simulink model "armModelLQG"  (R2018b)
settings: Solver=ode15s  StartTime=0.0  StopTime=10  MaxStep=1e-4  RelTol=1e-6  AbsTol=1e-7
values from neighbouring files (symbols this model uses):
  Cv1 = 1.3*10^(-6)*60/(2*pi)    (= 1.24140855612e-05)    [setup.m]
  Cv2 = 1.3*10^(-6)*60/(2*pi)    (= 1.24140855612e-05)    [setup.m]
  Cv3 = 1.3*10^(-6)*60/(2*pi)    (= 1.24140855612e-05)    [setup.m]
  effWorm = 0.8    [setup.m]
  J1 = 1.3*10^(-4)    (= 0.00013)    [setup.m]
  J2 = 0.79*10^(-4)    (= 7.9e-05)    [setup.m]
  J3 = 0.98*10^(-4)    (= 9.8e-05)    [setup.m]
  Ke1 = 0.15    [setup.m]
  Ke2 = 0.12    [setup.m]
  Ke3 = 0.12    [setup.m]
  Km1 = 0.15    [setup.m]
  Km2 = 0.12    [setup.m]
  Km3 = 0.12    [setup.m]
  N1 = 36    [setup.m]
  N2 = 36    [setup.m]
  N3 = 36    [setup.m]
  R1 = 1.9    [setup.m]
  R2 = 2.45    [setup.m]
  R3 = 1.9    [setup.m]
undefined symbols (not defined in the file or in its folder): A, B, C, Continuous, D, Time, X, Y, Z
libraries: sm_lib x92, nesl_utility x26, simulink x5, Parts_Lib x2, Contact_Forces_Lib x2, ctrlSharedLib x1
(part 4 of 4)

== system armModelLQG/ARM plant /Pop Transform4 1 ==
  Rotational fix1 : sm_lib/Frames and Transforms/Rigid Transform  TranslationMethod=None  TranslationStandardOffset=0  TranslationLengthUnit=m  TranslationStandardAxis=+Z  TranslationCartesianOffset=[0 0 0]  TranslationROffset=0  TranslationROffsetUnits=m  TranslationZOffset=0  TranslationZOffsetUnits=m  TranslationThetaOffset=0  TranslationThetaOffsetUnits=deg  RotationMethod=StandardAxis  RotationAngleUnits=deg  RotationStandardAxis=-Y  RotationAngle=90  RotationArbitraryAxis=[0 0 1]  FollAlignAxisA=+X  BaseAlignAxisA=+Y  FollAlignAxisB=+Y  BaseAlignAxisB=+Z  RotationSequenceAxes=FollowerAxes  RotationSequence=XYX  RotationSequenceAngles=[0 0 0]  RotationSequenceAnglesUnits=deg  RotationMatrix=[1 0 0; 0 1 0; 0 0 1]
  Rotational fix2 : sm_lib/Frames and Transforms/Rigid Transform  TranslationMethod=None  TranslationStandardOffset=0  TranslationLengthUnit=m  TranslationStandardAxis=+Z  TranslationCartesianOffset=[0 0 0]  TranslationROffset=0  TranslationROffsetUnits=m  TranslationZOffset=0  TranslationZOffsetUnits=m  TranslationThetaOffset=0  TranslationThetaOffsetUnits=deg  RotationMethod=StandardAxis  RotationAngleUnits=deg  RotationStandardAxis=-X  RotationAngle=90  RotationArbitraryAxis=[0 0 1]  FollAlignAxisA=+X  BaseAlignAxisA=+Y  FollAlignAxisB=+Y  BaseAlignAxisB=+Z  RotationSequenceAxes=FollowerAxes  RotationSequence=XYX  RotationSequenceAngles=[0 0 0]  RotationSequenceAnglesUnits=deg  RotationMatrix=[1 0 0; 0 1 0; 0 0 1]
  "Transform X " : sm_lib/Frames and Transforms/Rigid Transform  TranslationMethod=StandardAxis  TranslationStandardOffset=67.6  TranslationLengthUnit=mm  TranslationStandardAxis=-X  TranslationCartesianOffset=[0 0 -188]  TranslationROffset=0  TranslationROffsetUnits=m  TranslationZOffset=0  TranslationZOffsetUnits=m  TranslationThetaOffset=0  TranslationThetaOffsetUnits=deg  RotationMethod=None  RotationAngleUnits=deg  RotationStandardAxis=+Y  RotationAngle=90  RotationArbitraryAxis=[0 0 1]  FollAlignAxisA=+X  BaseAlignAxisA=+Y  FollAlignAxisB=+Y  BaseAlignAxisB=+Z  RotationSequenceAxes=FollowerAxes  RotationSequence=XYX  RotationSequenceAngles=[0 0 0]  RotationSequenceAnglesUnits=deg  RotationMatrix=[1 0 0; 0 1 0; 0 0 1]
  Transform y : sm_lib/Frames and Transforms/Rigid Transform  TranslationMethod=StandardAxis  TranslationStandardOffset=-447.93  TranslationLengthUnit=mm  TranslationStandardAxis=-Y  TranslationCartesianOffset=[0 0 -188]  TranslationROffset=0  TranslationROffsetUnits=m  TranslationZOffset=0  TranslationZOffsetUnits=m  TranslationThetaOffset=0  TranslationThetaOffsetUnits=deg  RotationMethod=None  RotationAngleUnits=deg  RotationStandardAxis=+Y  RotationAngle=90  RotationArbitraryAxis=[0 0 1]  FollAlignAxisA=+X  BaseAlignAxisA=+Y  FollAlignAxisB=+Y  BaseAlignAxisB=+Z  RotationSequenceAxes=FollowerAxes  RotationSequence=XYX  RotationSequenceAngles=[0 0 0]  RotationSequenceAnglesUnits=deg  RotationMatrix=[1 0 0; 0 1 0; 0 0 1]
  Transform z : sm_lib/Frames and Transforms/Rigid Transform  TranslationMethod=StandardAxis  TranslationStandardOffset=0.59  TranslationLengthUnit=mm  TranslationStandardAxis=-Z  TranslationCartesianOffset=[0 0 -188]  TranslationROffset=0  TranslationROffsetUnits=m  TranslationZOffset=0  TranslationZOffsetUnits=m  TranslationThetaOffset=0  TranslationThetaOffsetUnits=deg  RotationMethod=None  RotationAngleUnits=deg  RotationStandardAxis=+Y  RotationAngle=90  RotationArbitraryAxis=[0 0 1]  FollAlignAxisA=+X  BaseAlignAxisA=+Y  FollAlignAxisB=+Y  BaseAlignAxisB=+Z  RotationSequenceAxes=FollowerAxes  RotationSequence=XYX  RotationSequenceAngles=[0 0 0]  RotationSequenceAnglesUnits=deg  RotationMatrix=[1 0 0; 0 1 0; 0 0 1]
  Conn1 : PMIOPort  Side=Left
  Conn2 : PMIOPort  Port=2  Side=Right
  connections:
  Rotational fix1/RConn1 -- Conn2/RConn1
  Transform z/RConn1 -- Rotational fix1/LConn1
  Rotational fix2/RConn1 -- "Transform X "/LConn1
  Transform y/LConn1 -- "Transform X "/RConn1
  Transform z/LConn1 -- Transform y/RConn1
  Conn1/RConn1 -- Rotational fix2/LConn1

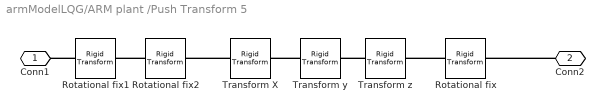
== system armModelLQG/ARM plant /Push Transform 5 ==
  Rotational fix : sm_lib/Frames and Transforms/Rigid Transform  TranslationMethod=None  TranslationStandardOffset=0  TranslationLengthUnit=m  TranslationStandardAxis=+Z  TranslationCartesianOffset=[0 0 0]  TranslationROffset=0  TranslationROffsetUnits=m  TranslationZOffset=0  TranslationZOffsetUnits=m  TranslationThetaOffset=0  TranslationThetaOffsetUnits=deg  RotationMethod=StandardAxis  RotationAngleUnits=deg  RotationStandardAxis=+X  RotationAngle=90  RotationArbitraryAxis=[0 0 1]  FollAlignAxisA=+X  BaseAlignAxisA=+Y  FollAlignAxisB=+Y  BaseAlignAxisB=+Z  RotationSequenceAxes=FollowerAxes  RotationSequence=XYX  RotationSequenceAngles=[0 0 0]  RotationSequenceAnglesUnits=deg  RotationMatrix=[1 0 0; 0 1 0; 0 0 1]
  Rotational fix1 : sm_lib/Frames and Transforms/Rigid Transform  TranslationMethod=None  TranslationStandardOffset=0  TranslationLengthUnit=m  TranslationStandardAxis=+Z  TranslationCartesianOffset=[0 0 0]  TranslationROffset=0  TranslationROffsetUnits=m  TranslationZOffset=0  TranslationZOffsetUnits=m  TranslationThetaOffset=0  TranslationThetaOffsetUnits=deg  RotationMethod=StandardAxis  RotationAngleUnits=deg  RotationStandardAxis=+Y  RotationAngle=-90  RotationArbitraryAxis=[0 0 1]  FollAlignAxisA=+X  BaseAlignAxisA=+Y  FollAlignAxisB=+Y  BaseAlignAxisB=+Z  RotationSequenceAxes=FollowerAxes  RotationSequence=XYX  RotationSequenceAngles=[0 0 0]  RotationSequenceAnglesUnits=deg  RotationMatrix=[1 0 0; 0 1 0; 0 0 1]
  Rotational fix2 : sm_lib/Frames and Transforms/Rigid Transform  TranslationMethod=None  TranslationStandardOffset=0  TranslationLengthUnit=m  TranslationStandardAxis=+Z  TranslationCartesianOffset=[0 0 0]  TranslationROffset=0  TranslationROffsetUnits=m  TranslationZOffset=0  TranslationZOffsetUnits=m  TranslationThetaOffset=0  TranslationThetaOffsetUnits=deg  RotationMethod=StandardAxis  RotationAngleUnits=deg  RotationStandardAxis=+X  RotationAngle=0  RotationArbitraryAxis=[0 0 1]  FollAlignAxisA=+X  BaseAlignAxisA=+Y  FollAlignAxisB=+Y  BaseAlignAxisB=+Z  RotationSequenceAxes=FollowerAxes  RotationSequence=XYX  RotationSequenceAngles=[0 0 0]  RotationSequenceAnglesUnits=deg  RotationMatrix=[1 0 0; 0 1 0; 0 0 1]
  "Transform X " : sm_lib/Frames and Transforms/Rigid Transform  TranslationMethod=StandardAxis  TranslationStandardOffset=18.98  TranslationLengthUnit=mm  TranslationStandardAxis=+X  TranslationCartesianOffset=[0 0 -188]  TranslationROffset=0  TranslationROffsetUnits=m  TranslationZOffset=0  TranslationZOffsetUnits=m  TranslationThetaOffset=0  TranslationThetaOffsetUnits=deg  RotationMethod=None  RotationAngleUnits=deg  RotationStandardAxis=+Y  RotationAngle=90  RotationArbitraryAxis=[0 0 1]  FollAlignAxisA=+X  BaseAlignAxisA=+Y  FollAlignAxisB=+Y  BaseAlignAxisB=+Z  RotationSequenceAxes=FollowerAxes  RotationSequence=XYX  RotationSequenceAngles=[0 0 0]  RotationSequenceAnglesUnits=deg  RotationMatrix=[1 0 0; 0 1 0; 0 0 1]
  Transform y : sm_lib/Frames and Transforms/Rigid Transform  TranslationMethod=StandardAxis  TranslationStandardOffset=-11.18  TranslationLengthUnit=mm  TranslationStandardAxis=+Y  TranslationCartesianOffset=[0 0 -188]  TranslationROffset=0  TranslationROffsetUnits=m  TranslationZOffset=0  TranslationZOffsetUnits=m  TranslationThetaOffset=0  TranslationThetaOffsetUnits=deg  RotationMethod=None  RotationAngleUnits=deg  RotationStandardAxis=+Y  RotationAngle=90  RotationArbitraryAxis=[0 0 1]  FollAlignAxisA=+X  BaseAlignAxisA=+Y  FollAlignAxisB=+Y  BaseAlignAxisB=+Z  RotationSequenceAxes=FollowerAxes  RotationSequence=XYX  RotationSequenceAngles=[0 0 0]  RotationSequenceAnglesUnits=deg  RotationMatrix=[1 0 0; 0 1 0; 0 0 1]
  Transform z : sm_lib/Frames and Transforms/Rigid Transform  TranslationMethod=StandardAxis  TranslationStandardOffset=-10  TranslationLengthUnit=mm  TranslationStandardAxis=+Z  TranslationCartesianOffset=[0 0 -188]  TranslationROffset=0  TranslationROffsetUnits=m  TranslationZOffset=0  TranslationZOffsetUnits=m  TranslationThetaOffset=0  TranslationThetaOffsetUnits=deg  RotationMethod=None  RotationAngleUnits=deg  RotationStandardAxis=+Y  RotationAngle=90  RotationArbitraryAxis=[0 0 1]  FollAlignAxisA=+X  BaseAlignAxisA=+Y  FollAlignAxisB=+Y  BaseAlignAxisB=+Z  RotationSequenceAxes=FollowerAxes  RotationSequence=XYX  RotationSequenceAngles=[0 0 0]  RotationSequenceAnglesUnits=deg  RotationMatrix=[1 0 0; 0 1 0; 0 0 1]
  Conn1 : PMIOPort  Side=Left
  Conn2 : PMIOPort  Port=2  Side=Right
  connections:
  Conn2/RConn1 -- Rotational fix/RConn1
  Rotational fix/LConn1 -- Transform z/RConn1
  "Transform X "/LConn1 -- Rotational fix2/RConn1
  Transform y/LConn1 -- "Transform X "/RConn1
  Transform z/LConn1 -- Transform y/RConn1
  Rotational fix1/LConn1 -- Conn1/RConn1
  Rotational fix2/LConn1 -- Rotational fix1/RConn1

== system armModelLQG/ARM plant /Push Transform1  ==
  Rotational fix : sm_lib/Frames and Transforms/Rigid Transform  TranslationMethod=None  TranslationStandardOffset=0  TranslationLengthUnit=m  TranslationStandardAxis=+Z  TranslationCartesianOffset=[0 0 0]  TranslationROffset=0  TranslationROffsetUnits=m  TranslationZOffset=0  TranslationZOffsetUnits=m  TranslationThetaOffset=0  TranslationThetaOffsetUnits=deg  RotationMethod=StandardAxis  RotationAngleUnits=deg  RotationStandardAxis=+Y  RotationAngle=-90  RotationArbitraryAxis=[0 0 1]  FollAlignAxisA=+X  BaseAlignAxisA=+Y  FollAlignAxisB=+Y  BaseAlignAxisB=+Z  RotationSequenceAxes=FollowerAxes  RotationSequence=XYX  RotationSequenceAngles=[0 0 0]  RotationSequenceAnglesUnits=deg  RotationMatrix=[1 0 0; 0 1 0; 0 0 1]
  "Transform Y 1 " : sm_lib/Frames and Transforms/Rigid Transform  TranslationMethod=StandardAxis  TranslationStandardOffset=-29  TranslationLengthUnit=mm  TranslationStandardAxis=+Y  TranslationCartesianOffset=[0 0 0]  TranslationROffset=0  TranslationROffsetUnits=m  TranslationZOffset=0  TranslationZOffsetUnits=m  TranslationThetaOffset=0  TranslationThetaOffsetUnits=deg  RotationMethod=None  RotationAngleUnits=deg  RotationStandardAxis=+Y  RotationAngle=90  RotationArbitraryAxis=[0 0 1]  FollAlignAxisA=+X  BaseAlignAxisA=+Y  FollAlignAxisB=+Y  BaseAlignAxisB=+Z  RotationSequenceAxes=FollowerAxes  RotationSequence=XYX  RotationSequenceAngles=[0 0 0]  RotationSequenceAnglesUnits=deg  RotationMatrix=[1 0 0; 0 1 0; 0 0 1]
  "Transform Z 1 " : sm_lib/Frames and Transforms/Rigid Transform  TranslationMethod=StandardAxis  TranslationStandardOffset=-32  TranslationLengthUnit=mm  TranslationStandardAxis=+Z  TranslationCartesianOffset=[0 0 0]  TranslationROffset=0  TranslationROffsetUnits=m  TranslationZOffset=0  TranslationZOffsetUnits=m  TranslationThetaOffset=0  TranslationThetaOffsetUnits=deg  RotationMethod=None  RotationAngleUnits=deg  RotationStandardAxis=+Y  RotationAngle=90  RotationArbitraryAxis=[0 0 1]  FollAlignAxisA=+X  BaseAlignAxisA=+Y  FollAlignAxisB=+Y  BaseAlignAxisB=+Z  RotationSequenceAxes=FollowerAxes  RotationSequence=XYX  RotationSequenceAngles=[0 0 0]  RotationSequenceAnglesUnits=deg  RotationMatrix=[1 0 0; 0 1 0; 0 0 1]
  Conn1 : PMIOPort  Side=Left
  Conn2 : PMIOPort  Port=2  Side=Right
  connections:
  "Transform Z 1 "/LConn1 -- "Transform Y 1 "/RConn1
  Conn2/RConn1 -- Rotational fix/RConn1
  Rotational fix/LConn1 -- "Transform Z 1 "/RConn1
  Conn1/RConn1 -- "Transform Y 1 "/LConn1

== system armModelLQG/ARM plant /Push Transform2  ==
  Rotational fix : sm_lib/Frames and Transforms/Rigid Transform  TranslationMethod=None  TranslationStandardOffset=0  TranslationLengthUnit=m  TranslationStandardAxis=+Z  TranslationCartesianOffset=[0 0 0]  TranslationROffset=0  TranslationROffsetUnits=m  TranslationZOffset=0  TranslationZOffsetUnits=m  TranslationThetaOffset=0  TranslationThetaOffsetUnits=deg  RotationMethod=StandardAxis  RotationAngleUnits=deg  RotationStandardAxis=+Y  RotationAngle=90  RotationArbitraryAxis=[0 0 1]  FollAlignAxisA=+X  BaseAlignAxisA=+Y  FollAlignAxisB=+Y  BaseAlignAxisB=+Z  RotationSequenceAxes=FollowerAxes  RotationSequence=XYX  RotationSequenceAngles=[0 0 0]  RotationSequenceAnglesUnits=deg  RotationMatrix=[1 0 0; 0 1 0; 0 0 1]
  "Transform X " : sm_lib/Frames and Transforms/Rigid Transform  TranslationMethod=StandardAxis  TranslationStandardOffset=-188  TranslationLengthUnit=mm  TranslationStandardAxis=+X  TranslationCartesianOffset=[0 0 -188]  TranslationROffset=0  TranslationROffsetUnits=m  TranslationZOffset=0  TranslationZOffsetUnits=m  TranslationThetaOffset=0  TranslationThetaOffsetUnits=deg  RotationMethod=None  RotationAngleUnits=deg  RotationStandardAxis=+Y  RotationAngle=90  RotationArbitraryAxis=[0 0 1]  FollAlignAxisA=+X  BaseAlignAxisA=+Y  FollAlignAxisB=+Y  BaseAlignAxisB=+Z  RotationSequenceAxes=FollowerAxes  RotationSequence=XYX  RotationSequenceAngles=[0 0 0]  RotationSequenceAnglesUnits=deg  RotationMatrix=[1 0 0; 0 1 0; 0 0 1]
  Conn1 : PMIOPort  Side=Left
  Conn2 : PMIOPort  Port=2  Side=Right
  connections:
  Conn2/RConn1 -- Rotational fix/RConn1
  Rotational fix/LConn1 -- "Transform X "/RConn1
  "Transform X "/LConn1 -- Conn1/RConn1

== system armModelLQG/ARM plant /Push Transform3  ==
  Rotational fix : sm_lib/Frames and Transforms/Rigid Transform  TranslationMethod=None  TranslationStandardOffset=0  TranslationLengthUnit=m  TranslationStandardAxis=+Z  TranslationCartesianOffset=[0 0 0]  TranslationROffset=0  TranslationROffsetUnits=m  TranslationZOffset=0  TranslationZOffsetUnits=m  TranslationThetaOffset=0  TranslationThetaOffsetUnits=deg  RotationMethod=StandardAxis  RotationAngleUnits=deg  RotationStandardAxis=+Y  RotationAngle=-90  RotationArbitraryAxis=[0 0 1]  FollAlignAxisA=+X  BaseAlignAxisA=+Y  FollAlignAxisB=+Y  BaseAlignAxisB=+Z  RotationSequenceAxes=FollowerAxes  RotationSequence=XYX  RotationSequenceAngles=[0 0 0]  RotationSequenceAnglesUnits=deg  RotationMatrix=[1 0 0; 0 1 0; 0 0 1]
  "Transform X " : sm_lib/Frames and Transforms/Rigid Transform  TranslationMethod=StandardAxis  TranslationStandardOffset=20  TranslationLengthUnit=mm  TranslationStandardAxis=+X  TranslationCartesianOffset=[0 0 -188]  TranslationROffset=0  TranslationROffsetUnits=m  TranslationZOffset=0  TranslationZOffsetUnits=m  TranslationThetaOffset=0  TranslationThetaOffsetUnits=deg  RotationMethod=None  RotationAngleUnits=deg  RotationStandardAxis=+Y  RotationAngle=90  RotationArbitraryAxis=[0 0 1]  FollAlignAxisA=+X  BaseAlignAxisA=+Y  FollAlignAxisB=+Y  BaseAlignAxisB=+Z  RotationSequenceAxes=FollowerAxes  RotationSequence=XYX  RotationSequenceAngles=[0 0 0]  RotationSequenceAnglesUnits=deg  RotationMatrix=[1 0 0; 0 1 0; 0 0 1]
  Transform y : sm_lib/Frames and Transforms/Rigid Transform  TranslationMethod=StandardAxis  TranslationStandardOffset=-0.22  TranslationLengthUnit=mm  TranslationStandardAxis=+Y  TranslationCartesianOffset=[0 0 -188]  TranslationROffset=0  TranslationROffsetUnits=m  TranslationZOffset=0  TranslationZOffsetUnits=m  TranslationThetaOffset=0  TranslationThetaOffsetUnits=deg  RotationMethod=None  RotationAngleUnits=deg  RotationStandardAxis=+Y  RotationAngle=90  RotationArbitraryAxis=[0 0 1]  FollAlignAxisA=+X  BaseAlignAxisA=+Y  FollAlignAxisB=+Y  BaseAlignAxisB=+Z  RotationSequenceAxes=FollowerAxes  RotationSequence=XYX  RotationSequenceAngles=[0 0 0]  RotationSequenceAnglesUnits=deg  RotationMatrix=[1 0 0; 0 1 0; 0 0 1]
  Transform z : sm_lib/Frames and Transforms/Rigid Transform  TranslationMethod=StandardAxis  TranslationStandardOffset=-215.5  TranslationLengthUnit=mm  TranslationStandardAxis=+Z  TranslationCartesianOffset=[0 0 -188]  TranslationROffset=0  TranslationROffsetUnits=m  TranslationZOffset=0  TranslationZOffsetUnits=m  TranslationThetaOffset=0  TranslationThetaOffsetUnits=deg  RotationMethod=None  RotationAngleUnits=deg  RotationStandardAxis=+Y  RotationAngle=90  RotationArbitraryAxis=[0 0 1]  FollAlignAxisA=+X  BaseAlignAxisA=+Y  FollAlignAxisB=+Y  BaseAlignAxisB=+Z  RotationSequenceAxes=FollowerAxes  RotationSequence=XYX  RotationSequenceAngles=[0 0 0]  RotationSequenceAnglesUnits=deg  RotationMatrix=[1 0 0; 0 1 0; 0 0 1]
  Conn1 : PMIOPort  Side=Left
  Conn2 : PMIOPort  Port=2  Side=Right
  connections:
  Conn2/RConn1 -- Rotational fix/RConn1
  Rotational fix/LConn1 -- Transform z/RConn1
  "Transform X "/LConn1 -- Conn1/RConn1
  Transform y/LConn1 -- "Transform X "/RConn1
  Transform z/LConn1 -- Transform y/RConn1

== system armModelLQG/ARM plant /Push Transform4  ==
  Rotational fix : sm_lib/Frames and Transforms/Rigid Transform  TranslationMethod=None  TranslationStandardOffset=0  TranslationLengthUnit=m  TranslationStandardAxis=+Z  TranslationCartesianOffset=[0 0 0]  TranslationROffset=0  TranslationROffsetUnits=m  TranslationZOffset=0  TranslationZOffsetUnits=m  TranslationThetaOffset=0  TranslationThetaOffsetUnits=deg  RotationMethod=StandardAxis  RotationAngleUnits=deg  RotationStandardAxis=+X  RotationAngle=90  RotationArbitraryAxis=[0 0 1]  FollAlignAxisA=+X  BaseAlignAxisA=+Y  FollAlignAxisB=+Y  BaseAlignAxisB=+Z  RotationSequenceAxes=FollowerAxes  RotationSequence=XYX  RotationSequenceAngles=[0 0 0]  RotationSequenceAnglesUnits=deg  RotationMatrix=[1 0 0; 0 1 0; 0 0 1]
  Rotational fix1 : sm_lib/Frames and Transforms/Rigid Transform  TranslationMethod=None  TranslationStandardOffset=0  TranslationLengthUnit=m  TranslationStandardAxis=+Z  TranslationCartesianOffset=[0 0 0]  TranslationROffset=0  TranslationROffsetUnits=m  TranslationZOffset=0  TranslationZOffsetUnits=m  TranslationThetaOffset=0  TranslationThetaOffsetUnits=deg  RotationMethod=StandardAxis  RotationAngleUnits=deg  RotationStandardAxis=+Y  RotationAngle=90  RotationArbitraryAxis=[0 0 1]  FollAlignAxisA=+X  BaseAlignAxisA=+Y  FollAlignAxisB=+Y  BaseAlignAxisB=+Z  RotationSequenceAxes=FollowerAxes  RotationSequence=XYX  RotationSequenceAngles=[0 0 0]  RotationSequenceAnglesUnits=deg  RotationMatrix=[1 0 0; 0 1 0; 0 0 1]
  "Transform X " : sm_lib/Frames and Transforms/Rigid Transform  TranslationMethod=StandardAxis  TranslationStandardOffset=67.6  TranslationLengthUnit=mm  TranslationStandardAxis=+X  TranslationCartesianOffset=[0 0 -188]  TranslationROffset=0  TranslationROffsetUnits=m  TranslationZOffset=0  TranslationZOffsetUnits=m  TranslationThetaOffset=0  TranslationThetaOffsetUnits=deg  RotationMethod=None  RotationAngleUnits=deg  RotationStandardAxis=+Y  RotationAngle=90  RotationArbitraryAxis=[0 0 1]  FollAlignAxisA=+X  BaseAlignAxisA=+Y  FollAlignAxisB=+Y  BaseAlignAxisB=+Z  RotationSequenceAxes=FollowerAxes  RotationSequence=XYX  RotationSequenceAngles=[0 0 0]  RotationSequenceAnglesUnits=deg  RotationMatrix=[1 0 0; 0 1 0; 0 0 1]
  Transform y : sm_lib/Frames and Transforms/Rigid Transform  TranslationMethod=StandardAxis  TranslationStandardOffset=-447.93  TranslationLengthUnit=mm  TranslationStandardAxis=+Y  TranslationCartesianOffset=[0 0 -188]  TranslationROffset=0  TranslationROffsetUnits=m  TranslationZOffset=0  TranslationZOffsetUnits=m  TranslationThetaOffset=0  TranslationThetaOffsetUnits=deg  RotationMethod=None  RotationAngleUnits=deg  RotationStandardAxis=+Y  RotationAngle=90  RotationArbitraryAxis=[0 0 1]  FollAlignAxisA=+X  BaseAlignAxisA=+Y  FollAlignAxisB=+Y  BaseAlignAxisB=+Z  RotationSequenceAxes=FollowerAxes  RotationSequence=XYX  RotationSequenceAngles=[0 0 0]  RotationSequenceAnglesUnits=deg  RotationMatrix=[1 0 0; 0 1 0; 0 0 1]
  Transform z : sm_lib/Frames and Transforms/Rigid Transform  TranslationMethod=StandardAxis  TranslationStandardOffset=0.59  TranslationLengthUnit=mm  TranslationStandardAxis=+Z  TranslationCartesianOffset=[0 0 -188]  TranslationROffset=0  TranslationROffsetUnits=m  TranslationZOffset=0  TranslationZOffsetUnits=m  TranslationThetaOffset=0  TranslationThetaOffsetUnits=deg  RotationMethod=None  RotationAngleUnits=deg  RotationStandardAxis=+Y  RotationAngle=90  RotationArbitraryAxis=[0 0 1]  FollAlignAxisA=+X  BaseAlignAxisA=+Y  FollAlignAxisB=+Y  BaseAlignAxisB=+Z  RotationSequenceAxes=FollowerAxes  RotationSequence=XYX  RotationSequenceAngles=[0 0 0]  RotationSequenceAnglesUnits=deg  RotationMatrix=[1 0 0; 0 1 0; 0 0 1]
  Conn1 : PMIOPort  Side=Left
  Conn2 : PMIOPort  Port=2  Side=Right
  connections:
  Conn2/RConn1 -- Rotational fix/RConn1
  Rotational fix/LConn1 -- Transform z/RConn1
  "Transform X "/LConn1 -- Rotational fix1/RConn1
  Transform y/LConn1 -- "Transform X "/RConn1
  Transform z/LConn1 -- Transform y/RConn1
  Rotational fix1/LConn1 -- Conn1/RConn1

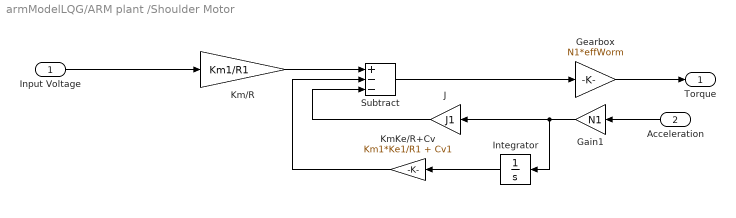
== system armModelLQG/ARM plant /Shoulder Motor  ==
  Input Voltage : Inport
  Acceleration : Inport  Port=2
  Gain1 : Gain  Gain=N1
  "Gearbox " : Gain  Gain=N1*effWorm
  Integrator : Integrator
  J : Gain  Gain=J1
  Km/R : Gain  Gain=Km1/R1
  KmKe/R+Cv : Gain  Gain=Km1*Ke1/R1 + Cv1
  Subtract : Sum  Inputs=+--
  "Torque " : Outport
  wires:
  Km/R/1 -> Subtract/1
  Subtract/1 -> "Gearbox "/1
  KmKe/R+Cv/1 -> Subtract/2
  "Gearbox "/1 -> "Torque "/1
  Acceleration/1 -> Gain1/1
  Input Voltage/1 -> Km/R/1
  Integrator/1 -> KmKe/R+Cv/1
  J/1 -> Subtract/3
  Gain1/1 -> Integrator/1, J/1

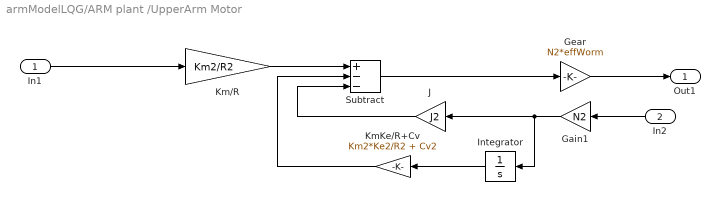
== system armModelLQG/ARM plant /UpperArm Motor ==
  In1 : Inport
  In2 : Inport  Port=2
  Gain1 : Gain  Gain=N2
  Gear : Gain  Gain=N2*effWorm
  Integrator : Integrator
  J : Gain  Gain=J2
  Km/R : Gain  Gain=Km2/R2
  KmKe/R+Cv : Gain  Gain=Km2*Ke2/R2 + Cv2
  Subtract : Sum  Inputs=+--
  Out1 : Outport
  wires:
  Km/R/1 -> Subtract/1
  Subtract/1 -> Gear/1
  KmKe/R+Cv/1 -> Subtract/2
  Gear/1 -> Out1/1
  In2/1 -> Gain1/1
  In1/1 -> Km/R/1
  Integrator/1 -> KmKe/R+Cv/1
  J/1 -> Subtract/3
  Gain1/1 -> Integrator/1, J/1

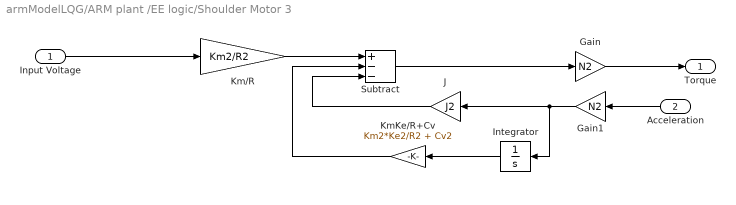
== system armModelLQG/ARM plant /EE logic/Shoulder Motor 3 ==
  Input Voltage : Inport
  Acceleration : Inport  Port=2
  Gain : Gain  Gain=N2
  Gain1 : Gain  Gain=N2
  Integrator : Integrator
  J : Gain  Gain=J2
  Km/R : Gain  Gain=Km2/R2
  KmKe/R+Cv : Gain  Gain=Km2*Ke2/R2 + Cv2
  Subtract : Sum  Inputs=+--
  "Torque " : Outport
  wires:
  Km/R/1 -> Subtract/1
  Subtract/1 -> Gain/1
  KmKe/R+Cv/1 -> Subtract/2
  Gain/1 -> "Torque "/1
  Acceleration/1 -> Gain1/1
  Input Voltage/1 -> Km/R/1
  Integrator/1 -> KmKe/R+Cv/1
  J/1 -> Subtract/3
  Gain1/1 -> Integrator/1, J/1

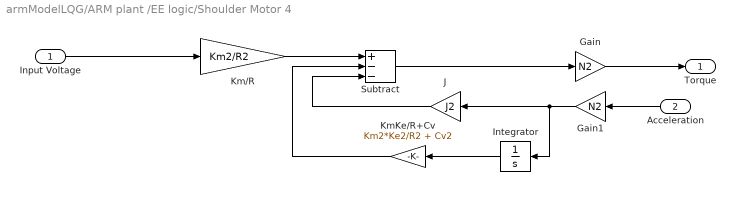
== system armModelLQG/ARM plant /EE logic/Shoulder Motor 4 ==
  Input Voltage : Inport
  Acceleration : Inport  Port=2
  Gain : Gain  Gain=N2
  Gain1 : Gain  Gain=N2
  Integrator : Integrator
  J : Gain  Gain=J2
  Km/R : Gain  Gain=Km2/R2
  KmKe/R+Cv : Gain  Gain=Km2*Ke2/R2 + Cv2
  Subtract : Sum  Inputs=+--
  "Torque " : Outport
  wires:
  Km/R/1 -> Subtract/1
  Subtract/1 -> Gain/1
  KmKe/R+Cv/1 -> Subtract/2
  Gain/1 -> "Torque "/1
  Acceleration/1 -> Gain1/1
  Input Voltage/1 -> Km/R/1
  Integrator/1 -> KmKe/R+Cv/1
  J/1 -> Subtract/3
  Gain1/1 -> Integrator/1, J/1

== matlab function armModelLQG/Ball Throw ==
  data: ballz input; y output
function y = fcn(ballz)
    %Function to do a waterfall throw
    %% init_________________________
    persistent counterIteration
    persistent counterTime
    persistent flag
    
    if isempty(flag)
        flag = 0;
    end
    if isempty(counterIteration)
        counterIteration = 1;
    end
    if isempty(counterTime)
        counterTime = 1;
    end
    ballCaughtThreshold = -0.31; % The plane where the ball is considered "caught"
    pattern = 1; %pattern 1 = waterfall, 2 = column
    
    if pattern == 1
        traj = [0 -0.06 -0.06 -0.06 -0.05 0 0.15 0;
            0 0 -0.1 -0.2 -0.3 0.2 0.1 0;
            0.00 0.00 -0.15 -0.4 -0.7 0.7 0.7 0];
    else
        traj = [0 -0.06 -0.06 -0.06 -0.05 0 0.15 0;
            -0 -0 -0 -0 -0 -0 -0 -0;
            0.00 0.00 -0.15 -0.4 -0.7 0.7 0.7 0];
    
    end
        %FOR COLS MAYBE    
        %traj = [-0.1 -0.05 0 0.15 0;
            %-0.15 -0.1 0 0.05 0;
            %-0.2 -0.7 0.7 0.7 0];
    %% Set flag ____________________
    if ballz < ballCaughtThreshold &&  ballz > -0.8 && flag == 0
        flag = 1;
    end
    if ballz < -0.8
        disp('BALL DROPPED RED TEAM WINS')
    end
    
    %% Iteration ___________________
    if flag == 0
        q_out = [0; 0; 0];
    else %flag = 1
        q_out = [traj(1,counterIteration); traj(2,counterIteration); traj(3,counterIteration)];
        counterIteration = counterIteration + 1;
        if counterIteration == length(traj) + 1
            counterIteration = 1;
            flag = 0;
        end
    end
y = [q_out; flag];

== matlab function armModelLQG/InverseKinematicLQR  ==
  data: q input size=3; state_trgt input size=3; output output double size=4 [..4]; flag input double size=1
function output = fcn(q, state_trgt, flag)
% Inverse kinematics function. See "setup.m" for source for H03 and J
%   *
% \[T]/
%input (q = initial/current state of [t1; t2; t3][rad], state_trget =
%target position of ee
%(x,y,z)[m], 
%global q_traj;
coder.extrinsic('exist') %needed to use exist in function block
final_size = 100; % Desired final vector length
persistent q_traj
persistent jteration
persistent q_traj_final
maxIterations = 15000;
reshaped_data2 = zeros(3,final_size); % Function block needs to pre define sizes of all variables
%retard = 0;
state_trgt(2) = state_trgt(2) - 0.03; %offset for the cup

%retard = exist('q_traj', 'var');
if isempty(q_traj)
    q_traj = zeros(3,maxIterations);
end
if isempty(jteration)
    jteration = 0;
end
if isempty(q_traj_final)
    q_traj_final = zeros(3,final_size);
end

%% ----- Idle section --------
%out = q;



%% Forward Kinematics part
% transformation matrix
if flag == 1 && jteration == 0
    H03 = @(theta1,theta2,theta3)  [ cos(theta1)*cos(theta2)*cos(theta3) - sin(theta1)*sin(theta3),   -cos(theta1)*sin(theta2),  -cos(theta3)*sin(theta1) - cos(theta1)*cos(theta2)*sin(theta3), (807*sin(theta1))/2000 + (cos(theta1)*cos(theta2))/50 - (3369*cos(theta1)*sin(theta2))/50000 - (44793*sin(theta1)*sin(theta3))/100000 + (44793*cos(theta1)*cos(theta2)*cos(theta3))/100000;
                                     cos(theta3)*sin(theta2),                                         cos(theta2),          -sin(theta2)*sin(theta3),                           (3369*cos(theta2))/50000 + sin(theta2)/50 + (44793*cos(theta3)*sin(theta2))/100000;
                                     cos(theta1)*sin(theta3) + cos(theta2)*cos(theta3)*sin(theta1),   -sin(theta1)*sin(theta2),  cos(theta1)*cos(theta3) - cos(theta2)*sin(theta1)*sin(theta3),  (cos(theta2)*sin(theta1))/50 - (807*cos(theta1))/2000 + (44793*cos(theta1)*sin(theta3))/100000 - (3369*sin(theta1)*sin(theta2))/50000 + (44793*cos(theta2)*cos(theta3)*sin(theta1))/100000;
                                     0,                                                               0,                0,                                          1];
    % Jacobian 
    J = @(theta1,theta2,theta3) [ (807*cos(theta1))/2000 - (cos(theta2)*sin(theta1))/50 - (44793*cos(theta1)*sin(theta3))/100000 + (3369*sin(theta1)*sin(theta2))/50000 - (44793*cos(theta2)*cos(theta3)*sin(theta1))/100000, - (3369*cos(theta1)*cos(theta2))/50000 - (cos(theta1)*sin(theta2))/50 - (44793*cos(theta1)*cos(theta3)*sin(theta2))/100000,  - (44793*cos(theta3)*sin(theta1))/100000 - (44793*cos(theta1)*cos(theta2)*sin(theta3))/100000;
                                   0,                                                                                                                                                                                         cos(theta2)/50 - (3369*sin(theta2))/50000 + (44793*cos(theta2)*cos(theta3))/100000,                                          -(44793*sin(theta2)*sin(theta3))/100000;
                                  (807*sin(theta1))/2000 + (cos(theta1)*cos(theta2))/50 - (3369*cos(theta1)*sin(theta2))/50000 - (44793*sin(theta1)*sin(theta3))/100000 + (44793*cos(theta1)*cos(theta2)*cos(theta3))/100000, - (3369*cos(theta2)*sin(theta1))/50000 - (sin(theta1)*sin(theta2))/50 - (44793*cos(theta3)*sin(theta1)*sin(theta2))/100000,  (44793*cos(theta1)*cos(theta3))/100000 - (44793*cos(theta2)*sin(theta1)*sin(theta3))/100000];

    %% optimization part
    % init for state ([x y z])
    H = H03(q(1),q(2),q(3));
    state = H(1:3,4);
    state_init = state;

    % Desired position in absolute coordinates relative to base [m]
    e = state_trgt - state;    % Error desried and actual pos

    % Maximum number of iterations
    %maxIterations = 15000;
    iterations = 1;

    % Error tolerance for final EE pos norm [m]
    tolerance = 0.01;
    stepsize = 1/5;    % Error stepsize for linearization

    % Coordinate initiation
    x = zeros(1,maxIterations); 
    y = zeros(1,maxIterations);
    z = zeros(1,maxIterations); 
    %global q_traj;
    q_traj = zeros(3,maxIterations);
    %data = zeros(3,maxIterations);

    % Levenberg Marquardt algorithm aims to solve the minimization problem
    % formulated as minimize(0.5*r'*We*r + 0.5*dQ'*Wn*dQ). Where dQ = Q(k+1) -
    % Q(k) and r = e - J'*dQ (e is the error we want to minimize). This means
    % that We is the cost-weight for the error and Wn is the cost-weight for
    % the angle change.

    % --- Weights and constraints ---
    % Error weight, specifies what error is prioritized to minimize [x y z]
    We = diag([1 1 1]);
    % Damping factor init. Updated in the loop as a function of the error.
    % Wn0 specifies weights for joint usage [Shoulder, upper arm, elbow]
    Wn0 = diag(1.2*[1.5 1 1]);
    % Joint limits (upper bound = lower bound) and joint limit weight
    JointLim = deg2rad([95 90 115]'); % [Shoulder, upper arm, elbow]
    Wl = diag(10*[1 1 1]);                          
    % --- Motion planning ---
    if norm(e) < tolerance
        % Do nothing if already within tolerance
        output = [q; 0];
        return
    end
    while norm(e) > tolerance
        % Current position calculations
        H = H03(q(1),q(2),q(3));
        state = H(1:3,4);

        q_traj(:,iterations) = q;
        
        Jacobian = J(q(1),q(2),q(3));   % Jacobian matrix

        %E = 0.5*diag(e')*We*diag(e);
        E = 0.5*e'*We*e*Wn0;
        Wn =  E + 2.5e-5*eye(3); % Wn = E + Wn_bias

        % ---------- Angle iteration ----------
        % Newton Raphson
        % q = q + Jacobian'*((desPos-curPos)/100);  % q(k+1) = q(k) + J'*e/step

        % Gauss Newton (NOT WORKING)
        % Jp = pinv(Jacobian);
        % gk = Jacobian'*We*((desPos-curPos)/1000);
        % q = q + Jp*gk;

        % Levenberg Marquardt
        lim = (diag(JointLim - abs(q)))'*Wl*(diag(JointLim - abs(q)));
        Hj = Jacobian'*We*Jacobian + Wn + lim^-1;
        gk = Jacobian'*We*((state_trgt-state)*stepsize);
        q = q + Hj^-1*gk;    % q(k+1) = q(k) + (J'We + Wn + lim^-1)^-1*J'We*e
        % q = q + (Jacobian'*We*Jacobian + Wn + ((diag(JointLim - abs(q)))'...
        %    *Wl*(diag(JointLim - abs(q))))^-1)^-1*(Jacobian'*We*...
        %    ((state_trgt-state)/100));
        % -------------------------------------

        % Error
        e = state_trgt - state;

        % Break Condition for max number of iterations
        if iterations >= maxIterations
            disp('BreakCondReached')
            break;
        end
        iterations = iterations + 1;
    end
    % EE vector trim
    x = x(1:iterations-1); y = y(1:iterations-1); z = z(1:iterations-1);
    q_traj_trimmed = q_traj(:,1:iterations-1);
    % ---------- Vector size reshaping ----------
    %final_size = 100; % Desired final vector length, defined at top of
    %funciton
    %data = q_traj;
    %disp(q_traj_trimmed);
    [dataRows dataCols] = size(q_traj_trimmed);
    data_size = q_traj_trimmed;
    n = ceil(length(data_size)/final_size);
    reshaped_data = zeros(size(data_size,1),round(length(data_size)/n));
    for row = 1:size(data_size,1)
        data = q_traj_trimmed(row,:);
        counter = 1;
        for i = 1:n:length(data)-n+1
            reshaped_data(row,counter) = mean(data(i:i+n-1));
            counter = counter + 1;
        end
    end
    %disp(reshaped_data);
    
    if size(reshaped_data,2) < final_size
        for roww = 1:size(reshaped_data,1)
            for col = 1:length(reshaped_data)
                reshaped_data2(roww,col) = reshaped_data(roww, col);
            end
            reshaped_data2(roww,length(data)/n:final_size) = ...
                reshaped_data(roww,length(data)/n);
        end
    end

    q_traj_final = reshaped_data2; % Reshaped trajectory data
    %q_out = q_traj(:,end);
    jteration = jteration+1;
end
%% ----- Display section -----


if jteration > 0
    out = q_traj_final(1:3,jteration); % NEEDS TO BE SET "1:3" instead of ":" (all the rows), otherwise it will think it has vAriAbLe sIzE
    jteration = jteration+1;
    %pause(0.001);
    if jteration == final_size
        jteration = 0;
    end
else
    out = q_traj_final(1:3,100);
end


%% ------- output -------------
%output = [0; 0; 0; 0;];
output = [out; jteration];

== matlab function armModelLQG/Trajectory Estimator ==
  data: ballPos input; y output
function y = fcn(ballPos)
    %% Init
    persistent x_intersect
    persistent y_intersect
    persistent dataPointer
    
    persistent ballTraj
    persistent ballTrajX
    
    persistent ballTrajY
    persistent ballTrajZ
    persistent stateFlag  %flag determining the state. 1 idle (ball being thrown) 2 record
    persistent catchFlag %Flag to send to activate linLqr
    
    % Number of sample points for estimating target.
    z_threshold = -0.15; % At which height is the ball considered "in the air"? [m]
    lengthSample = 20; % Number of points to guess ball position
    
    z_intercept = -0.4; % At which height will end effector catch the ball? [m]

    catchFlag = 0;
    
    if isempty(stateFlag)
        stateFlag = 1; %airFlag to signal the catch
    end
    if isempty(x_intersect)
        x_intersect = 0.4;
        y_intersect = 0;
        dataPointer = 1;
    end
    %fprintf("Waiting for throw...\n\n")        
    %data_ptr = 1;
    if isempty(ballTraj)
        ballTraj = zeros(3, lengthSample); %allocate maximum matrix size
        ballTrajX = zeros(1, lengthSample);
        ballTrajY = zeros(1, lengthSample);
        ballTrajZ = zeros(1, lengthSample);
    end
    %is_positive_direction_y = 0;
    %s_positive_direction_y = 0;
    

 
    %% Idle
    if stateFlag == 1 && ballPos(3) > z_threshold
        stateFlag = 2;
    end
    %data_array = 1:50;
    
    if stateFlag == 2 && dataPointer <= lengthSample
        ballTraj(:,dataPointer) = ballPos;
        if dataPointer == lengthSample
            stateFlag = 3;
            dataPointer = 0; %+1 gets added
        end
        dataPointer = dataPointer + 1;
    end
    
    if stateFlag == 3
        % Step 3: Fit a curve through the reflected points
        ballTrajX = ballTraj(1,:);
        ballTrajY = ballTraj(2,:);
        ballTrajZ = ballTraj(3,:);
        fit_xz_reflection = polyfit(ballTrajX', ballTrajZ', 2);
        fit_yz_reflection = polyfit(ballTrajY', ballTrajZ', 2);
        
        fit_xz_reflection(end) = fit_xz_reflection(end) - z_intercept;
        fit_yz_reflection(end) =  fit_yz_reflection(end) - z_intercept;
        rootsX = roots(fit_xz_reflection);
        rootsY = roots(fit_yz_reflection);
        
        
        %Determine the direction of ball throw
        if ballTrajX(1) < ballTrajX(end)
            is_positive_direction_x = 1;
        else
            is_positive_direction_x = 0;
        end

        if ballTrajY(1) < ballTrajY(end)
            is_positive_direction_y = 1;
        else
            is_positive_direction_y = 0;
        end
        
        %Check the direction of ball throw
        if is_positive_direction_x
            xIntersectC = max(rootsX);
            x_intersect = real(xIntersectC);
        else
            xIntersectC = min(rootsX);
            x_intersect = real(xIntersectC);
        end

        if is_positive_direction_y
            yIntersectC = max(rootsY);
            y_intersect = real(yIntersectC);
            %disp(xIntersectC);
        else
            yIntersectC = min(rootsY);
            y_intersect = real(yIntersectC);
            %disp(xIntersectC);
        end
        catchFlag = 1;
        stateFlag = 4;
    end
    
    if stateFlag == 4 && ballPos(3) <= z_threshold
        stateFlag = 1;
    end
    
    %disp(stateFlag);

y = [x_intersect, y_intersect, catchFlag];

== matlab function armModelLQG/Random Noise Gen ==
  data: u input; y output; t input
%Generates random noise with u as scalar
function y = fcn(u, t)

%y = u.*randn;
time = round(t)+1;
randVec1 = [1.0933 0.0774 -1.2141 -1.1135 -0.0068 1.5326 -0.7697 0.3714 -0.2256 1.1174 -1.0891'];
randVec2 = [0.0326 0.5525 1.1006 1.5442 0.0859 -1.4916 -0.7423 -1.0616 2.3505 -0.6156 0.7481]';
randVec3 = [-0.1924 0.8886 -0.7648 -1.4023 -1.4224 0.4882 -0.1774 -0.1961 1.4193 0.2916 0.1978]';

y = u.*[randVec1(time); randVec2(time); randVec3(time)];
